simulink model "sim12ex7"  (Simulink 4.00)
settings: Solver=ode23  SolverMode=SingleTasking  StartTime=0.0  StopTime=10  MaxStep=.050  RelTol=1e-3  AbsTol=1e-3
settings Model: LastModifiedBy=saadat  SaveTime=off  SaveOutput=off  LimitDataPoints=off  RTWTemplateMakefile=grt_vc.tmf  ExtModeTrigMode=oneshot  ExtModeArmWhenConnect=off

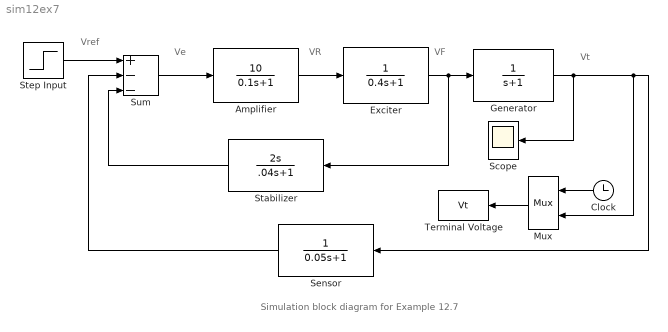
== system sim12ex7 ==
  note: Simulation block diagram for Example 12.7
  note: Vref
  note: Vt
  note: VF
  note: VR
  note: Ve
  Amplifier : TransferFcn  Numerator=[10]  Denominator="[0.1  1]"  AbsoluteTolerance=auto  Realization=auto
  Clock : Clock
      settings: DisplayTime=off  Decimation=10
  Exciter : TransferFcn  Numerator=[1]  Denominator="[0.4  1]"  AbsoluteTolerance=auto  Realization=auto
  Generator : TransferFcn  Numerator=[1]  Denominator="[1  1]"  AbsoluteTolerance=auto  Realization=auto
  Mux : Mux  Orientation=left  Inputs=2
      settings: DisplayOption=none
  Scope : Scope
      settings: TickLabels=on  TimeRange=10  YMin=0  YMax=1  SaveToWorkspace=off  SaveName=ScopeData  DataFormat=Array  LimitDataPoints=on  MaxDataPoints=5000
  Sensor : TransferFcn  Orientation=left  Numerator=[1]  Denominator="[0.05  1]"  AbsoluteTolerance=auto  Realization=auto
  Stabilizer : TransferFcn  Orientation=left  Numerator="[ 2  0]"  Denominator="[.04  1]"  AbsoluteTolerance=auto  Realization=auto
  Step Input : Step  Time=0  Before=0  After=1  SampleTime=0
  Sum : Sum  Inputs=+--  SaturateOnIntegerOverflow=on
  Terminal Voltage : ToWorkspace  VariableName=Vt  SampleTime=0  SaveFormat=Array
      settings: MaxDataPoints=1000
  wires:
  Mux/1 -> Terminal Voltage/1
  Clock/1 -> Mux/1
  Generator/1 -> Mux/2, Sensor/1, Scope/1
  Exciter/1 -> Stabilizer/1, Generator/1
  Sensor/1 -> Sum/2
  Stabilizer/1 -> Sum/3
  Amplifier/1 -> Exciter/1
  Sum/1 -> Amplifier/1
  Step Input/1 -> Sum/1
